simulink model "scene"  (R2021b)
settings: Solver=FixedStepAuto  StartTime=0.0  StopTime=6  FixedStep=1/25  MaxStep=1e-2  RelTol=1e-3
model workspace (MATLAB code in the model file):
  | a = [0 -0.425 -0.39225 0 0 0];
  | d = [0.089159 0 0 0.10915 0.09465 0.0823];
  | alpha = [pi/2 0 0 pi/2 -pi/2 0];
  | 
  | dhparams = [a' alpha' d' zeros(6,1)]
  | 
  | robot = rigidBodyTree;
  | 
  | body1 = rigidBody('body1');
  | jnt1 = rigidBodyJoint('jnt1','revolute');
  | body2 = rigidBody('body2');
  | jnt2 = rigidBodyJoint('jnt2','revolute');
  | body3 = rigidBody('body3');
  | jnt3 = rigidBodyJoint('jnt3','revolute');
  | body4 = rigidBody('body4');
  | jnt4 = rigidBodyJoint('jnt4','revolute');
  | body5 = rigidBody('body5');
  | jnt5 = rigidBodyJoint('jnt5','revolute');
  | body6 = rigidBody('body6');
  | jnt6 = rigidBodyJoint('jnt6','revolute');
  | 
  | setFixedTransform(jnt1,dhparams(1,:),'dh');
  | setFixedTransform(jnt2,dhparams(2,:),'dh');
  | setFixedTransform(jnt3,dhparams(3,:),'dh');
  | setFixedTransform(jnt4,dhparams(4,:),'dh');
  | setFixedTransform(jnt5,dhparams(5,:),'dh');
  | setFixedTransform(jnt6,dhparams(6,:),'dh');
  | 
  | body1.Joint = jnt1;
  | body2.Joint = jnt2;
  | body3.Joint = jnt3;
  | body4.Joint = jnt4;
  | body5.Joint = jnt5;
  | body6.Joint = jnt6;
  | 
  | addBody(robot,body1,'base')
  | addBody(robot,body2,'body1')
  | addBody(robot,body3,'body2')
  | addBody(robot,body4,'body3')
  | addBody(robot,body5,'body4')
  | addBody(robot,body6,'body5')
  | 
  | showdetails(robot)
  | show(robot)
values from neighbouring files (symbols this model uses):
  b_c = 0    [scene_parameters.m]
  b_lb = -0.5    [scene_parameters.m]
  b_ub = 1    [scene_parameters.m]
  D_o = [ (2*sqrt(mox*kox))*dr 0 0 ... (first row only)    [scene_parameters.m]
  D_p = [(2*sqrt(mpx*kpx))*dr 0 0 ... (first row only)    [scene_parameters.m]
  K_d_pd = eye(3)    [scene_parameters.m]
  k_n = -log((1+sensitivity_measure)/(1-sensitivity_measure))/pd_x_pdd_min    [scene_parameters.m]
  K_o = [kox 0 0 ... (first row only)    [scene_parameters.m]
  K_p = [kpx 0 0 ... (first row only)    [scene_parameters.m]
  k_p = -log((1-sensitivity_measure)/(1+sensitivity_measure))/pd_x_pdd_max    [scene_parameters.m]
  K_p_pd = eye(3)*4    [scene_parameters.m]
  M_o = [mox 0 0 ... (first row only)    [scene_parameters.m]
  M_p = [mpx 0 0 ... (first row only)    [scene_parameters.m]
libraries: robotmaniplib x7, dspinverses x3, robotcorelib x2, vrlib x2, matrix_library x1
settings Model: Creator=chsl  LastModifiedBy=jensh
settings SolverCC: AlgebraicLoopSolver=LineSearch
settings DataIOCC: ReturnWorkspaceOutputs=off
settings DebuggingCC: SFMachineParentedDataDiag=warning  ArithmeticOperatorsInVariantConditions=warning
settings SFSimCC: SimUseLocalCustomCode=off  CustomCodeUndefinedFunction=UseInterfaceOnly
settings RTWCC: RTWUseLocalCustomCode=off

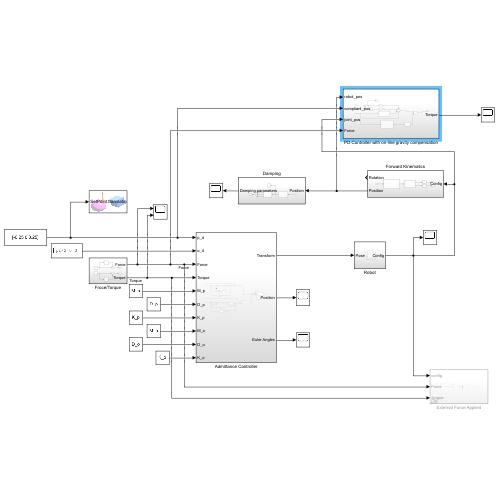
[thumbnail: Simulink's stored preview of the top-level diagram]
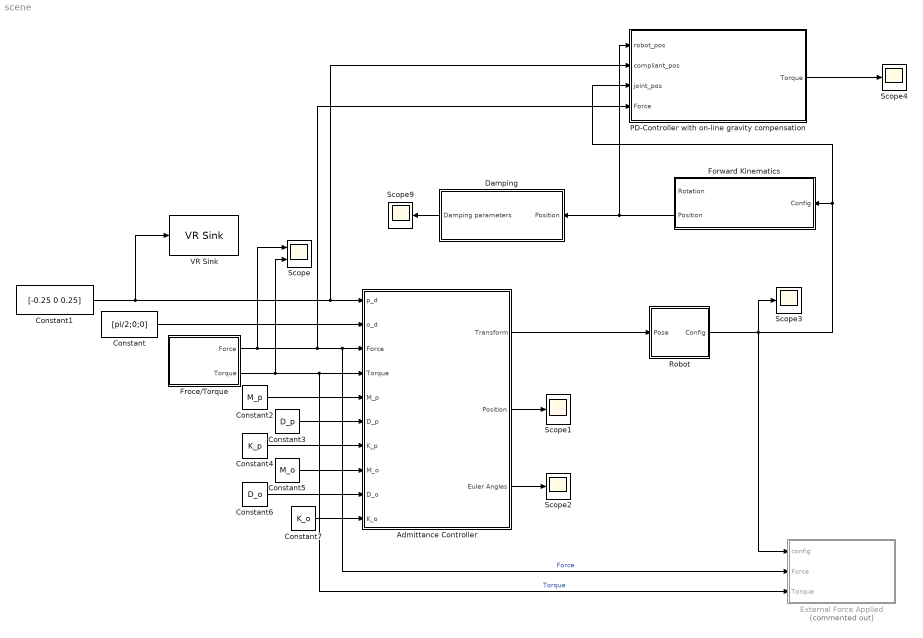
== system scene ==
  Admittance Controller : Subsystem
  Constant : Constant  Value=[pi/2;0;0]
  Constant1 : Constant  Value=[-0.25 0 0.25]
  Constant2 : Constant  Value=M_p
  Constant3 : Constant  Value=D_p
  Constant4 : Constant  Value=K_p
  Constant5 : Constant  Value=M_o
  Constant6 : Constant  Value=D_o
  Constant7 : Constant  Value=K_o
  Damping : Subsystem
  External Force Applied : Subsystem  Commented=on
  Forward Kinematics : Subsystem
  Froce/Torque : Subsystem
  PD-Controller with on-line gravity compensation : Subsystem
  Robot : Subsystem
  Scope : Scope  NumInputPorts=2
  Scope{1..4,9} (5 alike) : Scope
  VR Sink : vrlib/VR Sink  InstantiateOnLoad=on  SampleTime=-1  ViewEnable=on  RemoteChange=off  RemoteView=off  FieldsWritten=SetPoint.translation.3.1.1.double  WorldFileName=scene_environment.x3d  WorldDescription=Simple Robot Scene  AutoView=off  VideoDimensions=[]  AllowVariableSize=off
  wires:
  Froce/Torque/1(Force) -> Scope/1, PD-Controller with on-line gravity compensation/4(Force), External Force Applied/2(Force), Admittance Controller/3(Force)  "Force"
  Constant1/1 -> VR Sink/1, PD-Controller with on-line gravity compensation/2(compliant_pos), Admittance Controller/1(p_d)
  Froce/Torque/2(Torque) -> Scope/2, External Force Applied/3(Torque), Admittance Controller/4(Torque)  "Torque"
  Constant/1 -> Admittance Controller/2(o_d)
  Constant7/1 -> Admittance Controller/10(K_o)
  Constant6/1 -> Admittance Controller/9(D_o)
  Constant5/1 -> Admittance Controller/8(M_o)
  Constant4/1 -> Admittance Controller/7(K_p)
  Constant3/1 -> Admittance Controller/6(D_p)
  Constant2/1 -> Admittance Controller/5(M_p)
  Admittance Controller/2(Position) -> Scope1/1
  Admittance Controller/3(Euler Angles) -> Scope2/1
  Damping/1(Damping parameters) -> Scope9/1
  Robot/1(Config) -> Scope3/1, PD-Controller with on-line gravity compensation/3(joint_pos), Forward Kinematics/1(Config), External Force Applied/1(config)
  Admittance Controller/1(Transform) -> Robot/1(Pose)
  PD-Controller with on-line gravity compensation/1(Torque) -> Scope4/1
  Forward Kinematics/2(Position) -> PD-Controller with on-line gravity compensation/1(robot_pos), Damping/1(Position)

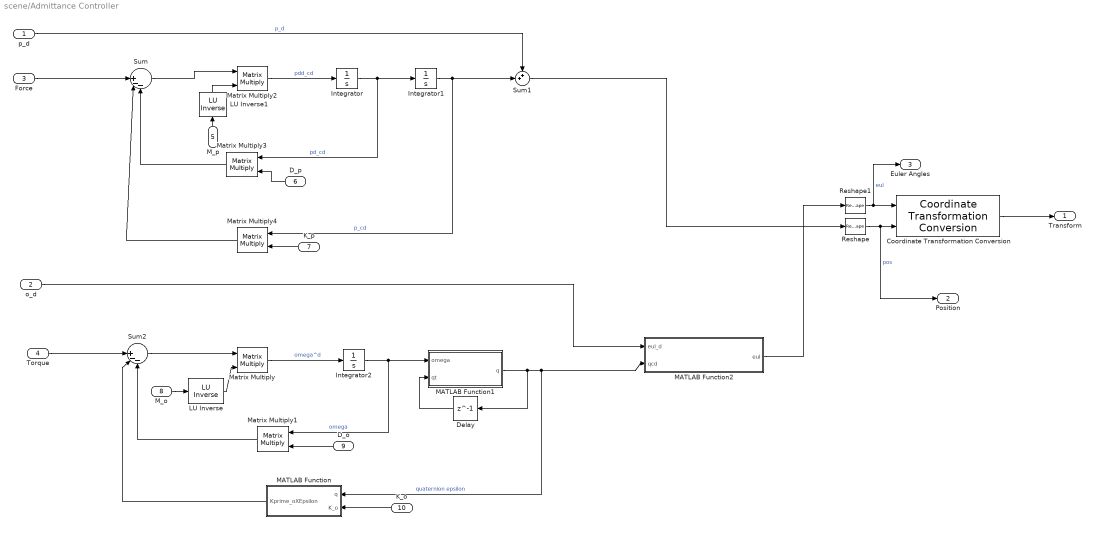
== system scene/Admittance Controller ==
  p_d : Inport
  o_d : Inport  Port=2
  Force : Inport  Port=3
  Torque : Inport  Port=4
  M_p : Inport  Port=5
  D_p : Inport  Port=6
  K_p : Inport  Port=7
  M_o : Inport  Port=8
  D_o : Inport  Port=9
  K_o : Inport  Port=10
  " LU Inverse" : dspinverses/ LU Inverse
  " LU Inverse1" : dspinverses/ LU Inverse
  Coordinate Transformation Conversion : robotcorelib/Coordinate Transformation Conversion  InputRepresentation=Euler Angles  InputEulerSequence=XYZ  ShowTrVecInputPort=on  OutputRepresentation=Homogeneous Transformation  OutputEulerSequence=ZYX  ShowTrVecOutputPort=on  SimulateUsing=Interpreted execution
      settings: SourceProductBaseCode=NV,RO,RR,UV
  Delay : Delay  DelayLength=1  InitialCondition=[1 0 0 0]
  Integrator : Integrator
  Integrator1 : Integrator
  Integrator2 : Integrator
  MATLAB Function : MATLAB Function  TreatAsAtomicUnit=on
  MATLAB Function1 : MATLAB Function  TreatAsAtomicUnit=on
  MATLAB Function2 : MATLAB Function  TreatAsAtomicUnit=on
  Matrix Multiply{,1..4} (5 alike) : Product  Multiplication=Matrix(*)
  Reshape : Reshape  OutputDimensionality=Column vector (2-D)
  Reshape1 : Reshape  OutputDimensionality=Column vector (2-D)
  Sum : Sum  Inputs=||+--
  Sum1 : Sum  Inputs=++|
  Sum2 : Sum  Inputs=||+--
  Transform : Outport
  Position : Outport  Port=2
  Euler Angles : Outport  Port=3
  wires:
  Force/1 -> Sum/1
  Integrator/1 -> Matrix Multiply3/1, Integrator1/1  "pd_cd"
  Integrator1/1 -> Matrix Multiply4/1, Sum1/2  "p_cd"
  p_d/1 -> Sum1/1  "p_d"
  Matrix Multiply3/1 -> Sum/3
  Matrix Multiply4/1 -> Sum/2
  Sum/1 -> Matrix Multiply2/1
  Matrix Multiply2/1 -> Integrator/1  "pdd_cd"
  Torque/1 -> Sum2/1
  Sum2/1 -> Matrix Multiply/1
  Matrix Multiply/1 -> Integrator2/1  "omega^d"
  Integrator2/1 -> Matrix Multiply1/1, MATLAB Function1/1(omega)  "omega"
  Matrix Multiply1/1 -> Sum2/3
  MATLAB Function1/1(q) -> Delay/1, MATLAB Function/1(q), MATLAB Function2/2(qcd)  "quaternion epsilon"
  K_o/1 -> MATLAB Function/2(K_o)
  MATLAB Function/1(Kprime_oXEpsilon) -> Sum2/2
  Delay/1 -> MATLAB Function1/2(qt)
  o_d/1 -> MATLAB Function2/1(eul_d)
  " LU Inverse"/1 -> Matrix Multiply/2
  M_o/1 -> " LU Inverse"/1
  D_o/1 -> Matrix Multiply1/2
  " LU Inverse1"/1 -> Matrix Multiply2/2
  M_p/1 -> " LU Inverse1"/1
  D_p/1 -> Matrix Multiply3/2
  K_p/1 -> Matrix Multiply4/2
  Reshape1/1 -> Euler Angles/1, Coordinate Transformation Conversion/1  "eul"
  Reshape/1 -> Position/1, Coordinate Transformation Conversion/2  "pos"
  Coordinate Transformation Conversion/1 -> Transform/1
  MATLAB Function2/1(eul) -> Reshape1/1
  Sum1/1 -> Reshape/1

== system scene/Damping ==
  Position : Inport
  Damping Estimation : Subsystem
  Mux : Mux  Inputs=3
  Scope9 : Scope
  User Intent : Subsystem
  Damping parameters : Outport
  wires:
  User Intent/1(pd_x_pdd) -> Scope9/1, Damping Estimation/1(pd_x_pdd)
  Damping Estimation/3(b_r_z) -> Mux/3
  Position/1 -> User Intent/1(Position)
  Damping Estimation/1(b_r_x) -> Mux/1
  Damping Estimation/2(b_r_y) -> Mux/2
  Mux/1 -> Damping parameters/1

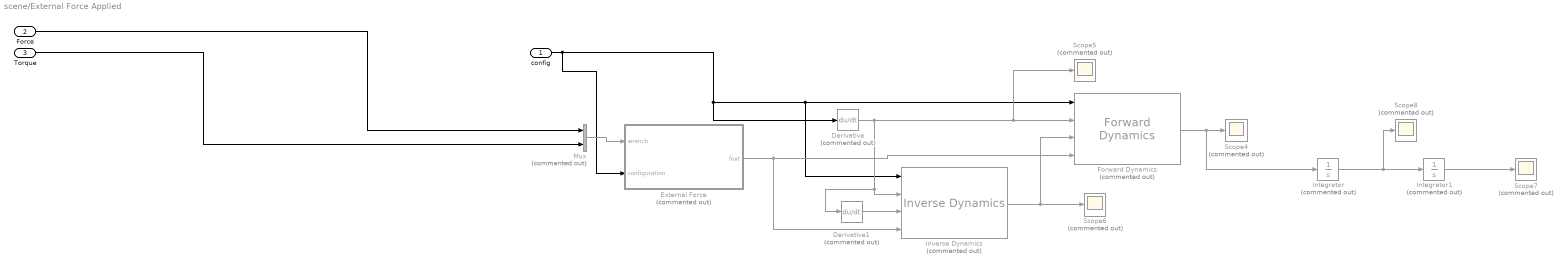
== system scene/External Force Applied ==
  config : Inport
  Force : Inport  Port=2
  Torque : Inport  Port=3
  Derivative : Derivative  Commented=on
  Derivative1 : Derivative  Commented=on
  External Force : MATLAB Function  Commented=on  TreatAsAtomicUnit=on
  Forward Dynamics : robotmaniplib/Forward Dynamics  Commented=on  RigidBodyTree=ur10_robot  SimulateUsing=Interpreted execution
  Integrator : Integrator  Commented=on
  Integrator1 : Integrator  Commented=on
  Inverse Dynamics : robotmaniplib/Inverse Dynamics  Commented=on  RigidBodyTree=ur10_robot  SimulateUsing=Interpreted execution
      settings: SourceProductBaseCode=RO
  Mux : Mux  Commented=on  Inputs=2
  Scope{4..8} (5 alike) : Scope  Commented=on
  wires:
  config/1 -> External Force/2(configuration), Derivative/1, Inverse Dynamics/1, Forward Dynamics/1
  Derivative/1 -> Derivative1/1, Inverse Dynamics/2, Scope5/1, Forward Dynamics/2
  Forward Dynamics/1 -> Integrator/1, Scope4/1
  External Force/1(fext) -> Inverse Dynamics/4, Forward Dynamics/4
  Integrator/1 -> Scope8/1, Integrator1/1
  Derivative1/1 -> Inverse Dynamics/3
  Integrator1/1 -> Scope7/1
  Inverse Dynamics/1 -> Forward Dynamics/3, Scope6/1
  Mux/1 -> External Force/1(wrench)
  Torque/1 -> Mux/2
  Force/1 -> Mux/1

== system scene/Forward Kinematics ==
  Config : Inport
  Coordinate Transformation Conversion : robotcorelib/Coordinate Transformation Conversion  InputRepresentation=Homogeneous Transformation  InputEulerSequence=ZYX  ShowTrVecInputPort=on  OutputRepresentation=Euler Angles  OutputEulerSequence=XYZ  ShowTrVecOutputPort=on  SimulateUsing=Interpreted execution
      settings: SourceProductBaseCode=NV,RO,RR,UV
  Get Transform : robotmaniplib/Get Transform  RigidBodyTree=ur10_robot  SourceBody=tool0  TargetBody=base_link  SimulateUsing=Interpreted execution
  Reshape : Reshape
  Reshape1 : Reshape
  Rotation : Outport
  Position : Outport  Port=2
  wires:
  Config/1 -> Get Transform/1
  Get Transform/1 -> Coordinate Transformation Conversion/1
  Reshape/1 -> Position/1
  Coordinate Transformation Conversion/2 -> Reshape/1
  Reshape1/1 -> Rotation/1
  Coordinate Transformation Conversion/1 -> Reshape1/1

== system scene/Froce//Torque ==
  Sum : Sum  Inputs=-+|
  Sum1 : Sum  Inputs=|+-
  Transport Delay : TransportDelay
  Transport Delay1 : TransportDelay
  f : Step  Before=[0 0 0]'  After=[1 -1/2 0]'  SampleTime=0
  tau : Step  Before=[0 0 0]'  After=[1 -1/2 0]'  SampleTime=0
  Force : Outport
  Torque : Outport  Port=2
  wires:
  Sum/1 -> Force/1
  tau/1 -> Transport Delay/1, Sum1/1
  Sum1/1 -> Torque/1
  Transport Delay/1 -> Sum1/2
  f/1 -> Transport Delay1/1, Sum/2
  Transport Delay1/1 -> Sum/1

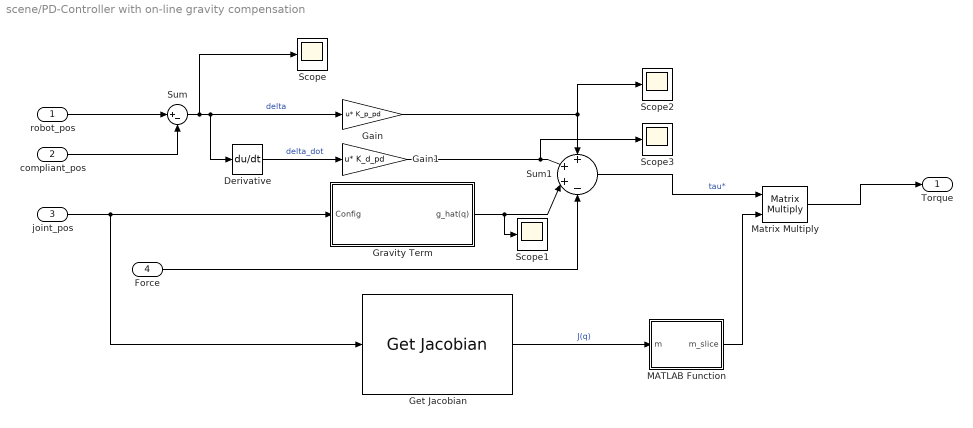
== system scene/PD-Controller with on-line gravity compensation ==
  robot_pos : Inport
  compliant_pos : Inport  Port=2
  joint_pos : Inport  Port=3
  Force : Inport  Port=4
  Derivative : Derivative
  Gain : Gain  Gain=K_p_pd  Multiplication=Matrix(u*K)
  Gain1 : Gain  Gain=K_d_pd  Multiplication=Matrix(u*K)
  Get Jacobian : robotmaniplib/Get Jacobian  RigidBodyTree=ur10_robot  EndEffector=tool0  SimulateUsing=Interpreted execution
      settings: SourceProductBaseCode=RO
  Gravity Term : Subsystem
  MATLAB Function : MATLAB Function  TreatAsAtomicUnit=on
  Matrix Multiply : Product  Multiplication=Matrix(*)
  Scope{,1..3} (4 alike) : Scope
  Sum : Sum  Inputs=|+-
  Sum1 : Sum  Inputs=+|+|+|-
  Torque : Outport
  wires:
  compliant_pos/1 -> Sum/2
  robot_pos/1 -> Sum/1
  Sum/1 -> Scope/1, Derivative/1, Gain/1  "delta"
  Force/1 -> Sum1/4
  Gain/1 -> Sum1/1, Scope2/1
  Gain1/1 -> Scope3/1, Sum1/2
  Derivative/1 -> Gain1/1  "delta_dot"
  joint_pos/1 -> Gravity Term/1(Config), Get Jacobian/1
  Gravity Term/1(g_hat(q)) -> Scope1/1, Sum1/3
  Sum1/1 -> Matrix Multiply/1  "tau*"
  Matrix Multiply/1 -> Torque/1
  Get Jacobian/1 -> MATLAB Function/1(m)  "J(q)"
  MATLAB Function/1(m_slice) -> Matrix Multiply/2

== system scene/Robot ==
  Pose : Inport
  Constant8 : Constant  Value=[0.25 0.25 0.25 1 1 1]
  Inverse Kinematics : robotmaniplib/Inverse Kinematics  RigidBodyTree=ur10_robot  EndEffector=tool0  ShowInfo=off  SolverName=BFGS Gradient Projection  EnforceJointLimits=on  MaxIterations=1500  MaxTime=10  GradientTolerance=1e-7  SolutionTolerance=1e-6  StepTolerance=1e-14  ErrorChangeTolerance=1e-12  UseErrorDamping=on  DampingBias=0.0025  SimulateUsing=Interpreted execution
  Unit Delay : UnitDelay  InitialCondition=zeros(6,1)  SampleTime=-1  HasFrameUpgradeWarning=on
  VR RigidBodyTree : vrlib/VR RigidBodyTree  VrmlFile=scene_environment.x3d  GroupNode=robot_parent  RBT=ur10_robot  useRBT=off  Ts=-1  ForceViewerOpen=off
      settings: SourceProductBaseCode=SL
  Config : Outport
  wires:
  Inverse Kinematics/1 -> VR RigidBodyTree/1, Config/1, Unit Delay/1
  Constant8/1 -> Inverse Kinematics/2  "Pose Weights"
  Pose/1 -> Inverse Kinematics/1
  Unit Delay/1 -> Inverse Kinematics/3

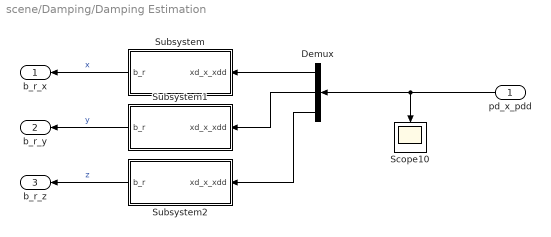
== system scene/Damping/Damping Estimation ==
  pd_x_pdd : Inport
  Demux : Demux  Outputs=3
  Scope10 : Scope
  Subsystem : Subsystem
  Subsystem1 : Subsystem
  Subsystem2 : Subsystem
  b_r_x : Outport
  b_r_y : Outport  Port=2
  b_r_z : Outport  Port=3
  wires:
  Subsystem/1(b_r) -> b_r_x/1  "x"
  Subsystem1/1(b_r) -> b_r_y/1  "y"
  Demux/1 -> Subsystem/1(xd_x_xdd)
  Demux/2 -> Subsystem1/1(xd_x_xdd)
  Subsystem2/1(b_r) -> b_r_z/1  "z"
  Demux/3 -> Subsystem2/1(xd_x_xdd)
  pd_x_pdd/1 -> Scope10/1, Demux/1

== system scene/Damping/User Intent ==
  Position : Inport
  Derivative2 : Derivative
  Derivative3 : Derivative
  MATLAB Function1 : MATLAB Function  TreatAsAtomicUnit=on
  Scope9 : Scope  NumInputPorts=3
  pd_x_pdd : Outport
  wires:
  Derivative3/1 -> MATLAB Function1/2(pdd), Scope9/1
  Position/1 -> Scope9/3, Derivative2/1
  Derivative2/1 -> MATLAB Function1/1(pd), Derivative3/1, Scope9/2
  MATLAB Function1/1(pd_x_pdd) -> pd_x_pdd/1

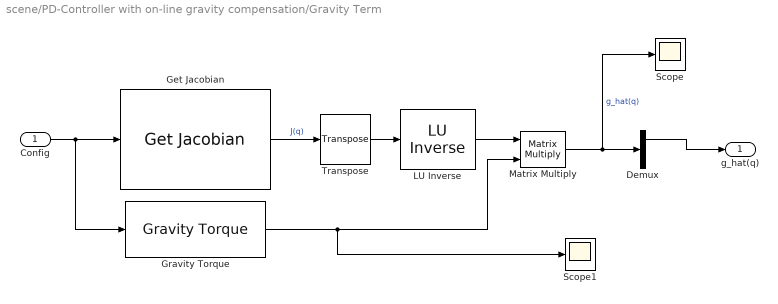
== system scene/PD-Controller with on-line gravity compensation/Gravity Term ==
  Config : Inport
  " LU Inverse" : dspinverses/ LU Inverse
  Demux : Demux  Outputs=2
  Get Jacobian : robotmaniplib/Get Jacobian  RigidBodyTree=ur10_robot  EndEffector=tool0  SimulateUsing=Interpreted execution
      settings: SourceProductBaseCode=RO
  Gravity Torque : robotmaniplib/Gravity Torque  RigidBodyTree=ur10_robot  SimulateUsing=Interpreted execution
  Matrix Multiply : Product  Multiplication=Matrix(*)
  Scope : Scope
  Scope1 : Scope
  Transpose : matrix_library/Transpose
      settings: SourceProductBaseCode=SL
  g_hat(q) : Outport
  wires:
  Config/1 -> Gravity Torque/1, Get Jacobian/1
  Get Jacobian/1 -> Transpose/1  "J(q)"
  Transpose/1 -> " LU Inverse"/1
  " LU Inverse"/1 -> Matrix Multiply/1
  Gravity Torque/1 -> Scope1/1, Matrix Multiply/2
  Matrix Multiply/1 -> Scope/1, Demux/1  "g_hat(q)"
  Demux/1 -> g_hat(q)/1

== system scene/Damping/Damping Estimation/Subsystem ==
  xd_x_xdd : Inport
  If : If  IfExpression=u1 >= 0
  If Action Subsystem : Subsystem  TreatAsAtomicUnit=on
  If Action Subsystem1 : Subsystem  TreatAsAtomicUnit=on
  Merge : Merge
  b_r : Outport
  wires:
  xd_x_xdd/1 -> If Action Subsystem1/1(pd_x_pdd), If Action Subsystem/1(pd_x_pdd), If/1
  If Action Subsystem1/1(Out1) -> Merge/2
  If/1 -> If Action Subsystem/Action
  If/2 -> If Action Subsystem1/Action
  Merge/1 -> b_r/1
  If Action Subsystem/1(Out1) -> Merge/1

== system scene/Damping/Damping Estimation/Subsystem1 ==
  xd_x_xdd : Inport
  If : If  IfExpression=u1 >= 0
  If Action Subsystem : Subsystem  TreatAsAtomicUnit=on
  If Action Subsystem1 : Subsystem  TreatAsAtomicUnit=on
  Merge : Merge
  b_r : Outport
  wires:
  xd_x_xdd/1 -> If Action Subsystem1/1(pd_x_pdd), If Action Subsystem/1(pd_x_pdd), If/1
  If Action Subsystem1/1(Out1) -> Merge/2
  If/1 -> If Action Subsystem/Action
  If/2 -> If Action Subsystem1/Action
  Merge/1 -> b_r/1
  If Action Subsystem/1(Out1) -> Merge/1

== system scene/Damping/Damping Estimation/Subsystem2 ==
  xd_x_xdd : Inport
  If : If  IfExpression=u1 >= 0
  If Action Subsystem : Subsystem  TreatAsAtomicUnit=on
  If Action Subsystem1 : Subsystem  TreatAsAtomicUnit=on
  Merge : Merge
  b_r : Outport
  wires:
  xd_x_xdd/1 -> If Action Subsystem1/1(pd_x_pdd), If Action Subsystem/1(pd_x_pdd), If/1
  If Action Subsystem1/1(Out1) -> Merge/2
  If/1 -> If Action Subsystem/Action
  If/2 -> If Action Subsystem1/Action
  Merge/1 -> b_r/1
  If Action Subsystem/1(Out1) -> Merge/1

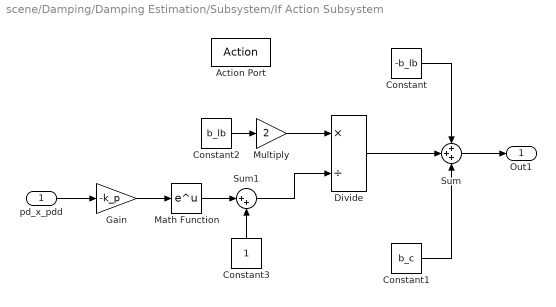
== system scene/Damping/Damping Estimation/Subsystem/If Action Subsystem ==
  pd_x_pdd : Inport
  Action Port : ActionPort  ActionPortLabel=if(u1 >= 0)
  Constant : Constant  Value=-b_lb
  Constant1 : Constant  Value=b_c
  Constant2 : Constant  Value=b_lb
  Constant3 : Constant
  Divide : Product  Inputs=*/
  Gain : Gain  Gain=-k_p
  Math Function : Math  SaturateOnIntegerOverflow=on
  Multiply : Gain  Gain=2
  Sum : Sum  Inputs=+++
  Sum1 : Sum  Inputs=|++
  Out1 : Outport
  wires:
  Sum/1 -> Out1/1
  Constant/1 -> Sum/1
  Constant1/1 -> Sum/3
  Divide/1 -> Sum/2
  Multiply/1 -> Divide/1
  Constant2/1 -> Multiply/1
  Sum1/1 -> Divide/2
  Constant3/1 -> Sum1/2
  Math Function/1 -> Sum1/1
  pd_x_pdd/1 -> Gain/1
  Gain/1 -> Math Function/1

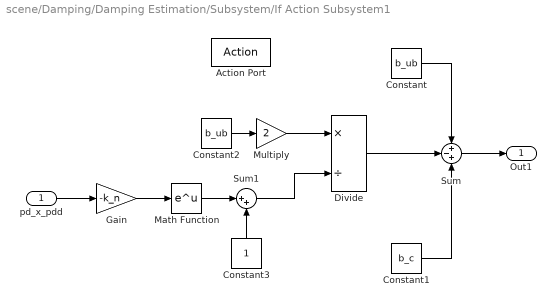
== system scene/Damping/Damping Estimation/Subsystem/If Action Subsystem1 ==
  pd_x_pdd : Inport
  Action Port : ActionPort  ActionPortLabel=else
  Constant : Constant  Value=b_ub
  Constant1 : Constant  Value=b_c
  Constant2 : Constant  Value=b_ub
  Constant3 : Constant
  Divide : Product  Inputs=*/
  Gain : Gain  Gain=-k_n
  Math Function : Math  SaturateOnIntegerOverflow=on
  Multiply : Gain  Gain=2
  Sum : Sum  Inputs=+-+
  Sum1 : Sum  Inputs=|++
  Out1 : Outport
  wires:
  Sum/1 -> Out1/1
  Constant/1 -> Sum/1
  Constant1/1 -> Sum/3
  Divide/1 -> Sum/2
  Multiply/1 -> Divide/1
  Constant2/1 -> Multiply/1
  Sum1/1 -> Divide/2
  Constant3/1 -> Sum1/2
  Math Function/1 -> Sum1/1
  pd_x_pdd/1 -> Gain/1
  Gain/1 -> Math Function/1

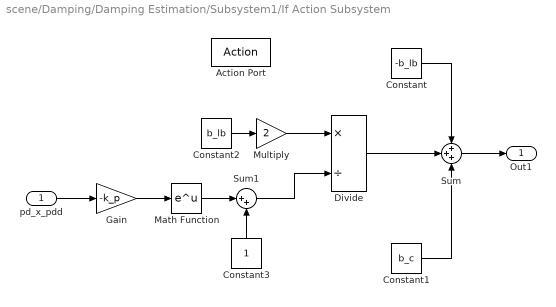
== system scene/Damping/Damping Estimation/Subsystem1/If Action Subsystem ==
  pd_x_pdd : Inport
  Action Port : ActionPort  ActionPortLabel=if(u1 >= 0)
  Constant : Constant  Value=-b_lb
  Constant1 : Constant  Value=b_c
  Constant2 : Constant  Value=b_lb
  Constant3 : Constant
  Divide : Product  Inputs=*/
  Gain : Gain  Gain=-k_p
  Math Function : Math  SaturateOnIntegerOverflow=on
  Multiply : Gain  Gain=2
  Sum : Sum  Inputs=+++
  Sum1 : Sum  Inputs=|++
  Out1 : Outport
  wires:
  Sum/1 -> Out1/1
  Constant/1 -> Sum/1
  Constant1/1 -> Sum/3
  Divide/1 -> Sum/2
  Multiply/1 -> Divide/1
  Constant2/1 -> Multiply/1
  Sum1/1 -> Divide/2
  Constant3/1 -> Sum1/2
  Math Function/1 -> Sum1/1
  pd_x_pdd/1 -> Gain/1
  Gain/1 -> Math Function/1

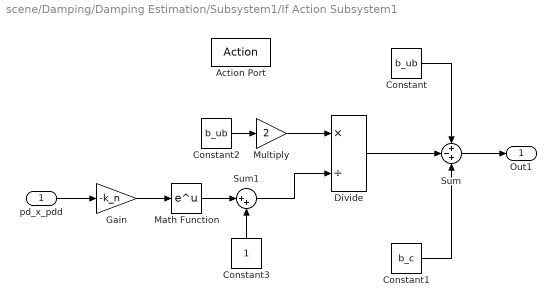
== system scene/Damping/Damping Estimation/Subsystem1/If Action Subsystem1 ==
  pd_x_pdd : Inport
  Action Port : ActionPort  ActionPortLabel=else
  Constant : Constant  Value=b_ub
  Constant1 : Constant  Value=b_c
  Constant2 : Constant  Value=b_ub
  Constant3 : Constant
  Divide : Product  Inputs=*/
  Gain : Gain  Gain=-k_n
  Math Function : Math  SaturateOnIntegerOverflow=on
  Multiply : Gain  Gain=2
  Sum : Sum  Inputs=+-+
  Sum1 : Sum  Inputs=|++
  Out1 : Outport
  wires:
  Sum/1 -> Out1/1
  Constant/1 -> Sum/1
  Constant1/1 -> Sum/3
  Divide/1 -> Sum/2
  Multiply/1 -> Divide/1
  Constant2/1 -> Multiply/1
  Sum1/1 -> Divide/2
  Constant3/1 -> Sum1/2
  Math Function/1 -> Sum1/1
  pd_x_pdd/1 -> Gain/1
  Gain/1 -> Math Function/1

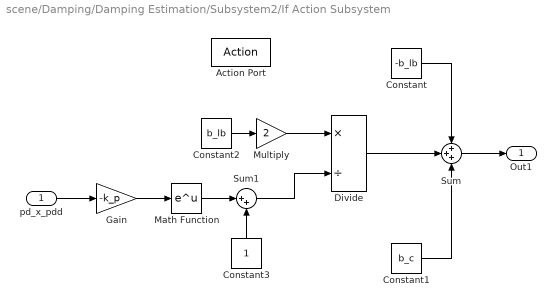
== system scene/Damping/Damping Estimation/Subsystem2/If Action Subsystem ==
  pd_x_pdd : Inport
  Action Port : ActionPort  ActionPortLabel=if(u1 >= 0)
  Constant : Constant  Value=-b_lb
  Constant1 : Constant  Value=b_c
  Constant2 : Constant  Value=b_lb
  Constant3 : Constant
  Divide : Product  Inputs=*/
  Gain : Gain  Gain=-k_p
  Math Function : Math  SaturateOnIntegerOverflow=on
  Multiply : Gain  Gain=2
  Sum : Sum  Inputs=+++
  Sum1 : Sum  Inputs=|++
  Out1 : Outport
  wires:
  Sum/1 -> Out1/1
  Constant/1 -> Sum/1
  Constant1/1 -> Sum/3
  Divide/1 -> Sum/2
  Multiply/1 -> Divide/1
  Constant2/1 -> Multiply/1
  Sum1/1 -> Divide/2
  Constant3/1 -> Sum1/2
  Math Function/1 -> Sum1/1
  pd_x_pdd/1 -> Gain/1
  Gain/1 -> Math Function/1

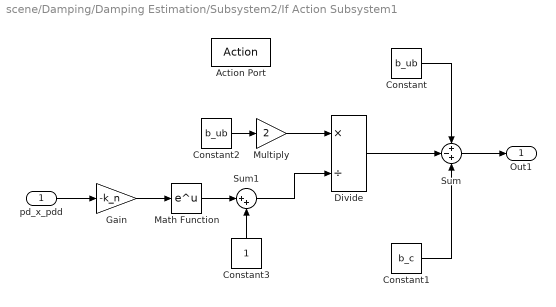
== system scene/Damping/Damping Estimation/Subsystem2/If Action Subsystem1 ==
  pd_x_pdd : Inport
  Action Port : ActionPort  ActionPortLabel=else
  Constant : Constant  Value=b_ub
  Constant1 : Constant  Value=b_c
  Constant2 : Constant  Value=b_ub
  Constant3 : Constant
  Divide : Product  Inputs=*/
  Gain : Gain  Gain=-k_n
  Math Function : Math  SaturateOnIntegerOverflow=on
  Multiply : Gain  Gain=2
  Sum : Sum  Inputs=+-+
  Sum1 : Sum  Inputs=|++
  Out1 : Outport
  wires:
  Sum/1 -> Out1/1
  Constant/1 -> Sum/1
  Constant1/1 -> Sum/3
  Divide/1 -> Sum/2
  Multiply/1 -> Divide/1
  Constant2/1 -> Multiply/1
  Sum1/1 -> Divide/2
  Constant3/1 -> Sum1/2
  Math Function/1 -> Sum1/1
  pd_x_pdd/1 -> Gain/1
  Gain/1 -> Math Function/1

== matlab function scene/External Force Applied/External Force ==
  settings: updateMethod=DISCRETE
  data: wrench input; fext output; configuration input

function fext = external_force(wrench, configuration)
persistent ur10_robot;
if isempty(ur10_robot)
    ur10_robot = ur10_robot_for_codegen("row");
end
fext_temp = externalForce(ur10_robot, "tool0", wrench, configuration);
if max(size(fext_temp)) ~= 11 || min(size(fext_temp)) ~= 6
    fext = zeros(6,10);
else
    fext = reshape(fext_temp, 6, 10);
end
end

== matlab function scene/Admittance Controller/MATLAB Function1 ==
  data: omega input; q output; qt input
function q = integration(omega, qt)
epsilon = [0 0 0 0];
qt = [qt(1) qt(2) qt(3) qt(4)];

dt = 1/500;

omega = omega * dt/2;

if norm(omega) > 0
    
    exp = [cos(norm(omega)); [omega/norm(omega)*sin(norm(omega))]'];

    epsilonQuat = quaternion(exp')*quaternion(qt);

    q = compact(epsilonQuat);
else
   q = qt; 
end

%We normalize to be safe
q = compact(normalize(quaternion(q)));

end

== matlab function scene/Admittance Controller/MATLAB Function2 ==
  data: eul_d input; qcd input; eul output
function eul = quaternion2eulerAngles(eul_d, qcd)



quat_qcd = quaternion(qcd);
quat_qcd = normalize(quat_qcd);

quat_qd = quaternion(eul2quat(eul_d'));
quat_qd = normalize(quat_qd);

qc = conj(quat_qcd * conj(quat_qd)); 


eul = quat2eul(compact(qc));

end

== matlab function scene/PD-Controller with on-line gravity compensation/MATLAB Function ==
  data: m input; m_slice output
function m_slice = matrix_slicer(m)
m_slice = m(1:3,:);
end

== matlab function scene/Damping/User Intent/MATLAB Function1 ==
  data: pd input; pd_x_pdd output; pdd input
function pd_x_pdd = user_intent(pd, pdd)
pd_x_pdd = pd.*pdd;
end

== matlab function scene/Admittance Controller/MATLAB Function ==
  data: q input; Kprime_oXEpsilon output; K_o input
function Kprime_oXEpsilon = ET(q, K_o)

S = [0 -q(4) q(3);
     q(4) 0 -q(2);
     -q(3) q(2) 0];

e = q(1)*eye(3)- S;

Kprime_o = 2*e'*K_o;

Kprime_oXEpsilon = Kprime_o * q(2:end)';

end
